simulink model "spacecraft4"  (R2019b)
settings: Solver=VariableStepAuto  StartTime=0.0  StopTime=10.0  RelTol=1e-3
model workspace (MAT data in the model file):
  A0 = [0  0  0  1  0  0; 0  0  0  0  1  0; 0  0  0  0  0  1; 0  0  0  0  0  0; 0  0  0  0  0  0; 0  0  0  0  0  0]
  I_x = Simulink.Parameter
  I_x.Value = 1.5
  I_x.DataType = 'auto'
  I_x.Dimensions = [1 1]
  I_y = Simulink.Parameter
  I_y.Value = 1.5
  I_y.DataType = 'auto'
  I_y.Dimensions = [1 1]
  d = Simulink.Parameter
  d.Value = 1
  d.DataType = 'auto'
  d.Dimensions = [1 1]
undefined symbols (not defined in the file or in its folder): Angle, Axis
libraries: vrlib x6, robotcorelib x1
settings Model: Creator=Tesla  LastModifiedBy=Tesla

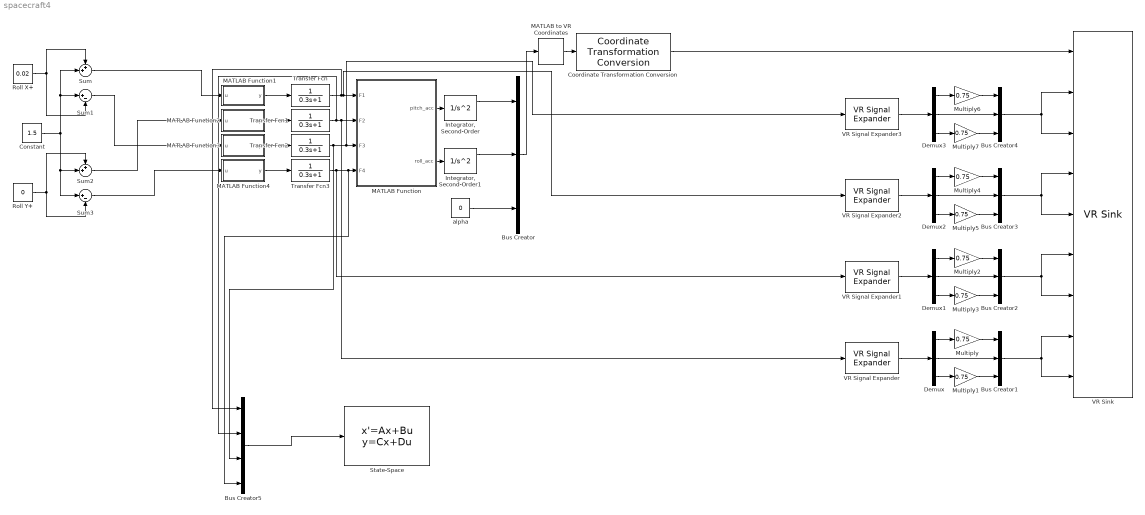
== system spacecraft4 ==
  Bus Creator{,1..4} (5 alike) : BusCreator  Inputs=3
  Bus Creator5 : BusCreator  Inputs=4
  Constant : Constant  Value=1.5
  Coordinate Transformation Conversion : robotcorelib/Coordinate Transformation Conversion  InputRepresentation=Euler Angles  InputEulerSequence=XYZ  ShowTrVecInputPort=on  OutputRepresentation=Axis-Angle  OutputEulerSequence=ZYX  ShowTrVecOutputPort=on  SimulateUsing=Interpreted execution
      settings: SourceProductBaseCode=RO
  Demux{,1..3} (4 alike) : Demux  Outputs=3
  "Integrator, Second-Order" : SecondOrderIntegrator
  "Integrator, Second-Order1" : SecondOrderIntegrator
  MATLAB Function : MATLAB Function  TreatAsAtomicUnit=on
  MATLAB Function1 : MATLAB Function  TreatAsAtomicUnit=on
  MATLAB Function2 : MATLAB Function  TreatAsAtomicUnit=on
  MATLAB Function3 : MATLAB Function  TreatAsAtomicUnit=on
  MATLAB Function4 : MATLAB Function  TreatAsAtomicUnit=on
  MATLAB to VR Coordinates : vrlib/Utilities/MATLAB to VR Coordinates
      settings: SourceProductName=Simulink  SourceProductBaseCode=SL
  Multiply{,1..7} (8 alike) : Gain  Gain=0.75
  Roll X+ : Constant  Value=0.02
  Roll Y+ : Constant  Value=0
  State-Space : StateSpace  InitialCondition=0
  Sum : Sum  Inputs=++|
  Sum1 : Sum  Inputs=|+-
  Sum2 : Sum  Inputs=++|
  Sum3 : Sum  Inputs=|+-
  Transfer Fcn{,1..3} (4 alike) : TransferFcn  Denominator=[0.3 1]
  VR Signal Expander{,1..3} (4 alike) : vrlib/VR Signal Expander  outwidth=3  outidx=[1 2 3]
      settings: SourceProductName=Simulink
  VR Sink : vrlib/VR Sink  InstantiateOnLoad=on  SampleTime=0.02  ViewEnable=on  RemoteChange=off  RemoteView=on  FieldsWritten=MB.rotation.4.1.1.double#Flame1.scale.3.1.1.double#Flame2.scale.3.1.1.double#Flame3.scale.3.1.1.double#Flame4.scale.3.1.1.double#Flame5.scale.3.1.1.double#Flame6.scale.3.1.1.double#Flame7.scale.3.1.1.double#Flame8.scale.3.1.1.double  WorldFileName=spacecraft4.wrl  AutoView=on  VideoDimensions=[]  AllowVariableSize=off  FigureProperties="{'Position', 'Name', 'Viewpoint', 'CameraBound', 'CameraDirection', 'CameraPosition', 'CameraUpVector', 'ZoomFactor', 'Antialiasing', 'Headlight', 'Lighting', 'NavPanel', 'Sound', 'StatusBar', 'Stereo3D', 'Stereo3DCameraOffset', 'Stereo3DHIT', 'ToolBar', 'Textures', 'Transparency', 'Triad', 'Wireframe', 'NavZones', 'NavMode', 'NavSpeed', 'CaptureFileFormat', 'CaptureFileName', 'Record2DCompressMethod', 'Record2DCompressQuality', 'Record2D', 'Record2DFileName', 'Record2DFPS'; [1.0000000000000000e+00   7.6000000000000000e+01   1.9200000000000000e+03   9.1300000000000000e+02], '', '_untitled_1', 'on', [4.7048804513036113e-01  -4.9427265429673733e-01  -7.3098258707240393e-01], [-8.1687564623843696e+02   8.5805285610059070e+02   2.6903178097575324e+02], [-3.2028911130800830e-01   6.7624230565538468e-01  -6.6340879495108274e-01], [1.0000000000000000e+00], 'on', 'on', 'on', 'halfbar', 'on', 'on', 'off', [1.0000000149011612e-01], [0.0000000000000000e+00], 'on', 'on', 'on', 'none', 'off', 'off', 'examine', 'veryfast', 'tif', '%f_anim_%n.tif', 'auto', [7.5000000000000000e+01], 'off', '%f_anim_%n.avi', 'auto'}"
      settings: SourceProductName=Simulink
  "alpha " : Constant  Value=0
  wires:
  MATLAB Function/1(pitch_acc) -> "Integrator, Second-Order"/1
  "Integrator, Second-Order"/1 -> Bus Creator/1
  Constant/1 -> Sum3/1, Sum2/2, Sum1/1, Sum/2
  Roll Y+/1 -> Sum3/2, Sum2/1
  Roll X+/1 -> Sum1/2, Sum/1
  Sum2/1 -> MATLAB Function2/1(u)
  Sum3/1 -> MATLAB Function4/1(u)
  VR Signal Expander/1 -> Demux/1
  MATLAB Function/2(roll_acc) -> "Integrator, Second-Order1"/1
  MATLAB to VR Coordinates/1 -> Coordinate Transformation Conversion/1
  "Integrator, Second-Order1"/1 -> Bus Creator/2
  "alpha "/1 -> Bus Creator/3
  Bus Creator/1 -> MATLAB to VR Coordinates/1
  Coordinate Transformation Conversion/1 -> VR Sink/1
  Demux/1 -> Multiply/1
  Multiply/1 -> Bus Creator1/1
  Multiply1/1 -> Bus Creator1/3
  Demux/3 -> Multiply1/1
  Demux/2 -> Bus Creator1/2
  Bus Creator1/1 -> VR Sink/9, VR Sink/8
  Multiply3/1 -> Bus Creator2/3
  Demux1/2 -> Bus Creator2/2
  Demux1/3 -> Multiply3/1
  Bus Creator2/1 -> VR Sink/7, VR Sink/6
  VR Signal Expander1/1 -> Demux1/1
  Multiply2/1 -> Bus Creator2/1
  Demux1/1 -> Multiply2/1
  Demux2/3 -> Multiply5/1
  Demux2/2 -> Bus Creator3/2
  Multiply4/1 -> Bus Creator3/1
  VR Signal Expander2/1 -> Demux2/1
  Sum/1 -> MATLAB Function1/1(u)
  Bus Creator3/1 -> VR Sink/4, VR Sink/5
  Demux2/1 -> Multiply4/1
  Multiply5/1 -> Bus Creator3/3
  Demux3/3 -> Multiply7/1
  Demux3/2 -> Bus Creator4/2
  Multiply6/1 -> Bus Creator4/1
  VR Signal Expander3/1 -> Demux3/1
  Sum1/1 -> MATLAB Function3/1(u)
  Bus Creator4/1 -> VR Sink/3, VR Sink/2
  Demux3/1 -> Multiply6/1
  Multiply7/1 -> Bus Creator4/3
  Transfer Fcn/1 -> Bus Creator5/1, VR Signal Expander2/1, MATLAB Function/1(F1)
  MATLAB Function1/1(y) -> Transfer Fcn/1
  MATLAB Function2/1(y) -> Transfer Fcn1/1
  Transfer Fcn1/1 -> Bus Creator5/2, VR Signal Expander/1, MATLAB Function/2(F2)
  MATLAB Function3/1(y) -> Transfer Fcn2/1
  Transfer Fcn2/1 -> VR Signal Expander3/1, MATLAB Function/3(F3), Bus Creator5/3
  MATLAB Function4/1(y) -> Transfer Fcn3/1
  Transfer Fcn3/1 -> VR Signal Expander1/1, Bus Creator5/4, MATLAB Function/4(F4)
  Bus Creator5/1 -> State-Space/1

== matlab function spacecraft4/MATLAB Function1 ==
  data: u input; y output
function y = fcn(u)

if u < 0
    y = 0;
else
    y = u
end
end

== matlab function spacecraft4/MATLAB Function ==
  data: F1 input; pitch_acc output; F2 input; F3 input; F4 input; roll_acc output
function [pitch_acc,roll_acc] = fcn(F1, F2, F3, F4)

d = 1;
Tx = d*(F2-F4);
Ty = d*(F1-F3);
Ix = 1.5
Iy = 1.5

pitch_acc = Ty/Iy
roll_acc = Tx/Ix

end

== matlab function spacecraft4/MATLAB Function2 ==
  data: u input; y output
function y = fcn(u)

if u < 0
    y = 0;
else
    y = u
end
end

== matlab function spacecraft4/MATLAB Function3 ==
  data: u input; y output
function y = fcn(u)

if u < 0
    y = 0;
else
    y = u
end
end

== matlab function spacecraft4/MATLAB Function4 ==
  data: u input; y output
function y = fcn(u)

if u < 0
    y = 0;
else
    y = u
end
end
